simulink model "orbit_simulator"  (R2023a)
settings: Solver=ode4  StartTime=0.0  StopTime=5700  FixedStep=0.1  RelTol=1e-3
undefined symbols (not defined in the file or in its folder): X, Y, Z
libraries: robotlib x7, sharedtransform x6, aerolibutil x4, sharedutil x1
settings Model: Creator=yhj2019  LastModifiedBy=ohminsik
settings OptimizationCC: EnhancedBackFolding=on  PassReuseOutputArgsThreshold=0  MaxStackSize=64  OptimizeBlockOrder=speed  DifferentSizesBufferReuse=on  OptimizationCustomize=off
settings DebuggingCC: ParameterTunabilityLossMsg=error
settings HardwareCC: ProdBitPerPointer=32  ProdBitPerSizeT=32  ProdBitPerPtrDiffT=32  ProdLargestAtomicFloat=None  ProdIntDivRoundTo=Undefined  ProdEndianess=Unspecified  ProdWordSize=32  ProdHWDeviceType=Generic->Unspecified (assume 32-bit Generic)  UseEmbeddedCoderFeatures=off
settings SFSimCC: MATLABDynamicMemAlloc=off
settings RTWCC: Description=Embedded Coder  SystemTargetFile=ert.tlc  HardwareBoard=Robot Operating System (ROS)  TLCOptions="-aInlineSetEventsForThisBaseRateFcn=TLC_FALSE -aSuppressMultiTaskScheduler=TLC_FALSE  -aRateBasedStepFcn=0"  TemplateMakefile=ert_default_tmf  Toolchain=Catkin  TargetLang=C++
settings CodeAppCC: ForceParamTrailComments=on  OperatorAnnotations=on
settings ERTTargetCC: ERTCustomFileBanners=off  SupportContinuousTime=on  SupportNonInlinedSFcns=on  RemoveResetFunc=off  ModelStepFunctionPrototypeControlCompliant=off

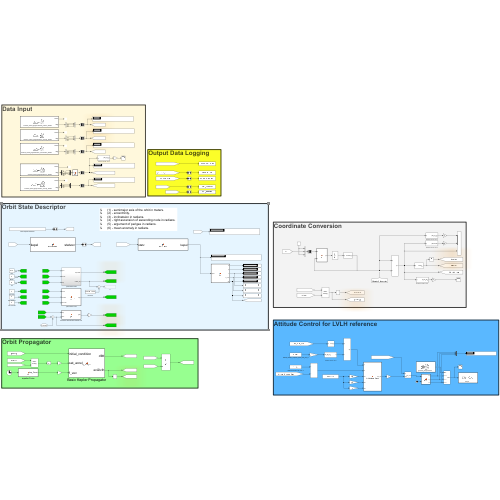
[thumbnail: Simulink's stored preview of the top-level diagram]
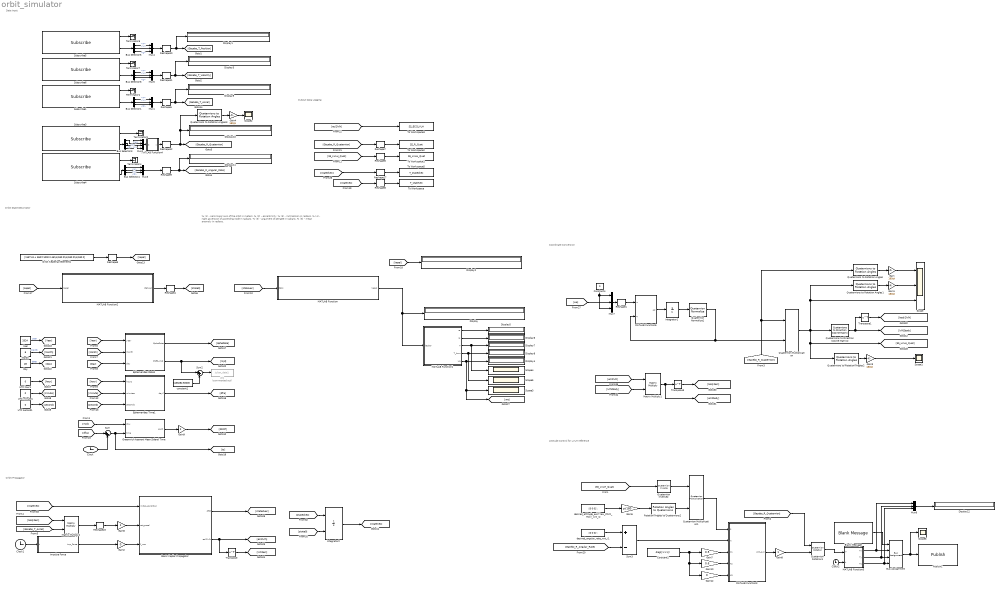
== system orbit_simulator ==
  note: Coordinate Conversion
  note: Orbit Propagator
  note: Output Data Logging
  note: Orbit State Descriptor
  note: Attitude Control for LVLH reference
  note: Data Input
  note: % (1) - semimajor axis of the orbit in meters.
      | % (2) - eccentricity.
      | % (3) - inclinatsion in radians.
      | % (4) - right ascension of ascending node in radians.
      | % (5) - argument of perigee in radians.
      | % (6) - mean anomaly in radians.
  Basic Kepler Propagator : MATLAB Function  TreatAsAtomicUnit=on
  Blank Message : robotlib/Blank Message  messageClass=Message  entityType=geometry_msgs/Vector3  messageType=geometry_msgs/Vector3  SampleTime=inf  legacyBusStruct=off
  Bus Assignment : BusAssignment  AssignedSignals=X,Y,Z
  Bus Selector{1,4..6} (4 alike) : BusSelector  OutputSignals=X,Y,Z
  Bus Selector3 : BusSelector  OutputSignals=X,Y,Z,W
  Clock : Clock
  Clock1 : Clock
  Clock2 : Clock
  Constant2 : Constant  Value=diag([1 1 1])
  Constant4 : Constant  Value=0
  Day : Constant  Value=28
  Display{,1..12} (13 alike) : Display
  Ephemerides Date1 : Subsystem
  Ephemerides Time1 : MATLAB Function  TreatAsAtomicUnit=on
  Gain{,1,3..4} (4 alike) : Gain  Gain=180/pi
  Gain10 : Gain  Gain=0.6
  Gain12 : Gain  Gain=0
  Gain2 : Gain  Gain=0
  Gain5 : Gain  Gain=pi/180
  Gain6 : Gain
  Gain7 : Gain  Gain=0.5
  Gain8 : Gain
  Gain9 : Gain
  Greenwich Aparent Mean Sideral Time : MATLAB Function  TreatAsAtomicUnit=on
  Impulse Force : MATLAB Function  TreatAsAtomicUnit=on
  Integrator1 : Integrator  InitialCondition=[1 0 0 0]'
  Integrator2 : Integrator  InitialConditionSource=external  InitialCondition=[-7000 0 0 0 -9.175045 0 5233.5]'
  JD1 : ToWorkspace  Commented=on  VariableName=Julian_date1  SampleTime=-1
  MATLAB Function : MATLAB Function  TreatAsAtomicUnit=on
  MATLAB Function1 : MATLAB Function  TreatAsAtomicUnit=on
  MATLAB Function2 : MATLAB Function  TreatAsAtomicUnit=on
  MATLAB Function3 : MATLAB Function  TreatAsAtomicUnit=on
  MATLAB Function4 : MATLAB Function  TreatAsAtomicUnit=on
  MATLAB Function5 : MATLAB Function  TreatAsAtomicUnit=on
  MATLAB Function6 : MATLAB Function  TreatAsAtomicUnit=on
  Matrix Multiply1 : Product  Multiplication=Matrix(*)
  Matrix Multiply2 : Product  Multiplication=Matrix(*)
  Month : Constant  Value=6
  Mux{1,3..7} (6 alike) : Mux  Inputs=3
  Mux2 : Mux
  Orbit Keplerian Elements : Constant  Value=[(6371.8 + 550)*1000 0 45*pi/180 0*pi/180 0*pi/180 0]
  Publish1 : robotlib/Publish  topicSource=Specify your own  topic=/torque  messageType=geometry_msgs/Vector3  legacyBusStruct=off  messageQueueLength=1
  Quaternion Inverse2 : aerolibutil/Quaternion Inverse
  Quaternion Multiplication : aerolibutil/Quaternion Multiplication
  Quaternion Multiplication1 : aerolibutil/Quaternion Multiplication
  Quaternion Normalize1 : sharedutil/Quaternion Normalize  aMode=aMode
  Quaternion Rotation1 : aerolibutil/Quaternion Rotation
  Quaternions to Direction Cosine Matrix2 : sharedtransform/Quaternions to  Direction Cosine Matrix  aMode=aMode
      settings: LibrarySourceBlock=|
      | aerolibtransform2/Quaternions to
      | Direction Cosine Matrix
  Quaternions to Rotation Angles : sharedtransform/Quaternions to Rotation Angles  rotationOrder=ZYX  aMode=aMode
  Quaternions to Rotation Angles1 : sharedtransform/Quaternions to Rotation Angles  rotationOrder=ZYX  aMode=aMode
  Quaternions to Rotation Angles2 : sharedtransform/Quaternions to Rotation Angles  rotationOrder=ZYX  aMode=aMode
  Quaternions to Rotation Angles3 : sharedtransform/Quaternions to Rotation Angles  rotationOrder=XYZ  aMode=aMode
  Reshape{1,5,9..12} (6 alike) : Reshape  OutputDimensionality=Column vector (2-D)
  Reshape{3..4,6..8,17} (6 alike) : Reshape  OutputDimensionality=Row vector (2-D)
  Reshape23 : Reshape  OutputDimensionality=Customize  OutputDimensions=[3,1]
  Rotation Angles to Quaternions2 : sharedtransform/Rotation Angles to Quaternions  rotationOrder=ZYX  aMode=aMode
  Scope : Scope  NumInputPorts=3
  Scope{1..6} (6 alike) : Scope
  Subscribe1 : robotlib/Subscribe  topicSource=Select from ROS network  topic=/reaction_wheel_plugin/transition_acceleration_throttle  messageType=geometry_msgs/Vector3  SampleTime=-1  legacyBusStruct=off  messageQueueLength=1
  Subscribe3 : robotlib/Subscribe  topicSource=Select from ROS network  topic=/reaction_wheel_plugin/quaternion_throttle  messageType=geometry_msgs/Quaternion  SampleTime=-1  legacyBusStruct=off  messageQueueLength=1
  Subscribe4 : robotlib/Subscribe  topicSource=Select from ROS network  topic=/reaction_wheel_plugin/rotation_velocity_throttle  messageType=geometry_msgs/Vector3  SampleTime=-1  legacyBusStruct=off  messageQueueLength=1
  Subscribe5 : robotlib/Subscribe  topicSource=Select from ROS network  topic=/reaction_wheel_plugin/transition_position_throttle  messageType=geometry_msgs/Vector3  SampleTime=-1  legacyBusStruct=off  messageQueueLength=1
  Subscribe6 : robotlib/Subscribe  topicSource=Select from ROS network  topic=/reaction_wheel_plugin/transition_velocity_throttle  messageType=geometry_msgs/Vector3  SampleTime=-1  legacyBusStruct=off  messageQueueLength=1
  Sum : Sum  Inputs=|++
  Sum2 : Sum  Inputs=|++
  Sum3 : Sum  Inputs=+-
  Terminator{1,3..4,6..7} (5 alike) : Terminator
  To Workspace : ToWorkspace  VariableName=T_statevec  SampleTime=-1
      settings: Save2DSignal=2-D array (concatenate along first dimension)
  To Workspace1 : ToWorkspace  VariableName=SS_LVLH_Quat  SampleTime=-1
      settings: Save2DSignal=2-D array (concatenate along first dimension)
  To Workspace2 : ToWorkspace  VariableName=SS_R_Quat  SampleTime=-1
      settings: Save2DSignal=2-D array (concatenate along first dimension)
  To Workspace3 : ToWorkspace  VariableName=SS_ECI2LVLH  SaveFormat=Structure With Time  SampleTime=-1
      settings: Save2DSignal=2-D array (concatenate along first dimension)
  To Workspace5 : ToWorkspace  VariableName=T_statedvec  SampleTime=-1
      settings: Save2DSignal=2-D array (concatenate along first dimension)
  Transpose : Math  Operator=transpose
  Transpose1 : Math  Operator=transpose
  Transpose3 : Math  Operator=transpose
  UTC hour1 : Constant  Value=0
  UTC minute1 : Constant  Value=0
  UTC second1 : Constant  Value=0
  Year : Constant  Value=2024
  constant1 : Constant  Value=2433282.50000
  desired_angular_rate_wrt_i1 : Constant  Value=[0 0 0]';
  desired_attitude_eulr(Yaw_Pitch_Roll)_wrt_i2 : Constant  Value=[0 0 0]';
  wires:
  MATLAB Function/1(kepel) -> Display/1, MATLAB Function1/1(kepler)
  Day/1 -> [Day]  "date"
  [statevec] -> Basic Kepler Propagator/1(initial_condition)
  Reshape3/1 -> [kepel]
  UTC hour1/1 -> [hour]
  Clock1/1 -> Impulse Force/1(t)
  MATLAB Function1/5(we) -> [we], Scope3/1, Display4/1
  Matrix Multiply2/1 -> Reshape23/1
  [minute] -> Ephemerides Time1/2(minutes)
  Reshape4/1 -> [state0]
  [statevec] -> Reshape8/1
  [kepel] -> MATLAB Function2/1(kepel)
  Clock/1 -> Sum/2
  MATLAB Function1/3(T) -> Scope4/1, Display7/1
  [Gazebo_T_Accel] -> Matrix Multiply2/2
  [statevec] -> MATLAB Function/1(statv)
  Basic Kepler Propagator/2(eci2lvlh) -> Transpose/1, [eci2lvlh]
  UTC minute1/1 -> [minute]
  Reshape8/1 -> To Workspace/1
  MATLAB Function1/1(ra) -> Display5/1
  [Year] -> Ephemerides Date1/1(year)
  [body2eci] -> Matrix Multiply2/1
  Month/1 -> [Month]  "month"
  Sum/1 -> Greenwich Aparent Mean Sideral Time/2(time), [ts]
  Basic Kepler Propagator/1(dfdt) -> [statedvec]
  Reshape17/1 -> To Workspace5/1
  [hour] -> Ephemerides Time1/1(hours)
  Gain6/1 -> Basic Kepler Propagator/2(sat_accel)
  MATLAB Function1/4(T_hour) -> Scope5/1, Display8/1
  Gain9/1 -> [GMST]
  Transpose/1 -> [lvlh2eci]
  [Month] -> Ephemerides Date1/2(month)
  Impulse Force/1(Imp_Force) -> Gain2/1
  MATLAB Function1/2(rp) -> Display6/1
  [Day] -> Ephemerides Date1/3(day)
  [statedvec] -> Reshape17/1
  [kepel] -> Display2/1
  UTC second1/1 -> [second]
  [second] -> Ephemerides Time1/3(seconds)
  [state0] -> Integrator2/2
  Sum2/1 -> JD1/1
  Gain2/1 -> Basic Kepler Propagator/3(f_vec)
  Ephemerides Date1/2(CNES_mdj) -> Sum2/1, [mjd]
  constant1/1 -> Sum2/2
  Reshape23/1 -> Gain6/1
  Integrator2/1 -> [statevec]
  Greenwich Aparent Mean Sideral Time/1(gwst) -> Gain9/1
  Ephemerides Date1/1(EpheDate) -> [EpheDate]
  Year/1 -> [Year]  "year"
  [statedvec] -> Integrator2/1
  MATLAB Function2/1(statvec) -> Reshape4/1
  Ephemerides Time1/1(dayf) -> [dfra]
  Orbit Keplerian Elements/1 -> Reshape3/1
  Subscribe5/2 -> Bus Selector5/1
  Bus Selector5/2 -> Mux4/2  "<Y>"
  Subscribe5/1 -> Terminator6/1
  Bus Selector5/3 -> Mux4/3  "<Z>"
  Bus Selector5/1 -> Mux4/1  "<X>"
  Mux4/1 -> Reshape10/1
  Reshape10/1 -> Display1/1, [Gazebo_T_Position]
  Bus Selector6/1 -> Mux5/1  "<X>"
  Bus Selector6/2 -> Mux5/2  "<Y>"
  Subscribe6/2 -> Bus Selector6/1
  Bus Selector6/3 -> Mux5/3  "<Z>"
  Subscribe6/1 -> Terminator7/1
  Mux5/1 -> Reshape11/1
  Reshape11/1 -> Display3/1, [Gazebo_T_Velocity]
  Bus Selector3/2 -> Mux2/3  "<Y>"
  Bus Selector3/4 -> Mux2/1  "<W>"
  Bus Selector3/1 -> Mux2/2  "<X>"
  Subscribe3/2 -> Bus Selector3/1
  Bus Selector3/3 -> Mux2/4  "<Z>"
  Subscribe3/1 -> Terminator3/1
  Mux2/1 -> MATLAB Function4/1(q)
  Bus Selector4/1 -> Mux3/1  "<X>"
  Mux3/1 -> Reshape9/1
  Bus Selector4/3 -> Mux3/3  "<Z>"
  Bus Selector4/2 -> Mux3/2  "<Y>"
  Subscribe4/1 -> Terminator4/1
  Subscribe4/2 -> Bus Selector4/1
  Reshape9/1 -> Display11/1, [Gazebo_R_Angular_Rate]
  Blank Message/1 -> Bus Assignment/1
  Bus Assignment/1 -> Scope6/1, Publish1/1
  Gain1/1 -> Scope/2
  Quaternion Multiplication/1 -> Quaternions to Direction Cosine Matrix2/1, [SS_LVLH_Quat], Quaternions to Rotation Angles2/1, Scope/3, Quaternions to Rotation Angles1/1
  Quaternion Normalize1/1 -> Quaternion Multiplication/2, MATLAB Function6/2(q)
  Quaternions to Rotation Angles1/1 -> Gain1/1
  Quaternions to Direction Cosine Matrix2/1 -> Transpose1/1, [lvlh2body]
  Quaternions to Rotation Angles/1 -> Gain/1
  Gain/1 -> Scope/1
  Transpose1/1 -> [body2lvlh]
  [Gazebo_R_Quaternion] -> Quaternion Multiplication/1, Quaternions to Rotation Angles/1
  MATLAB Function4/1(y) -> Reshape12/1
  Matrix Multiply1/1 -> Transpose3/1, [eci2body]
  Transpose3/1 -> [body2eci]
  [eci2lvlh] -> Matrix Multiply1/1
  [lvlh2body] -> Matrix Multiply1/2
  Subscribe1/2 -> Bus Selector1/1
  Subscribe1/1 -> Terminator1/1
  Bus Selector1/3 -> Mux1/3  "<Z>"
  Bus Selector1/1 -> Mux1/1  "<X>"
  Mux1/1 -> Reshape5/1
  Bus Selector1/2 -> Mux1/2  "<Y>"
  Reshape5/1 -> Display9/1, [Gazebo_T_Accel]
  Gain3/1 -> Scope1/1
  Quaternions to Rotation Angles2/1 -> Gain3/1
  Gain4/1 -> Scope2/1
  Quaternions to Rotation Angles3/1 -> Gain4/1
  Clock2/1 -> MATLAB Function5/2(t)
  MATLAB Function3/1(cntl_out) -> Gain8/1
  MATLAB Function5/3(Tz) -> Mux6/3, Bus Assignment/4
  MATLAB Function5/2(Ty) -> Mux6/2, Bus Assignment/3
  MATLAB Function5/1(Tx) -> Mux6/1, Bus Assignment/2
  Reshape6/1 -> To Workspace1/1
  [SS_LVLH_Quat] -> Reshape6/1
  [Gazebo_R_Quaternion] -> Reshape7/1
  Reshape7/1 -> To Workspace2/1
  [eci2lvlh] -> To Workspace3/1
  Reshape12/1 -> Quaternions to Rotation Angles3/1, Display10/1, [Gazebo_R_Quaternion]
  [Gazebo_R_Angular_Rate] -> Sum3/2
  Rotation Angles to Quaternions2/1 -> Quaternion Multiplication1/2
  Quaternion Inverse2/1 -> Quaternion Multiplication1/1
  Sum3/1 -> MATLAB Function3/2(w)
  Gain10/1 -> MATLAB Function3/4(K2)
  Gain7/1 -> MATLAB Function3/3(K1)
  Gain12/1 -> MATLAB Function3/5(K3)
  Constant2/1 -> Gain10/1, Gain12/1, Gain7/1
  Quaternion Multiplication1/1 -> MATLAB Function3/1(q)
  Gain5/1 -> Rotation Angles to Quaternions2/1
  desired_angular_rate_wrt_i1/1 -> Sum3/1
  desired_attitude_eulr(Yaw_Pitch_Roll)_wrt_i2/1 -> Gain5/1
  Constant4/1 -> Mux7/1, Mux7/3
  Reshape1/1 -> MATLAB Function6/1(w)
  Integrator1/1 -> Quaternion Normalize1/1
  MATLAB Function6/1(qd) -> Integrator1/1
  [we] -> Mux7/2
  Mux7/1 -> Reshape1/1
  [SS_LVLH_Quat] -> Quaternion Inverse2/1
  Gain8/1 -> Quaternion Rotation1/2
  Quaternion Rotation1/1 -> MATLAB Function5/1(T)
  [Gazebo_R_Quaternion] -> Quaternion Rotation1/1
  Mux6/1 -> Display12/1
  [mjd] -> Greenwich Aparent Mean Sideral Time/1(diju)
  [dfra] -> Sum/1

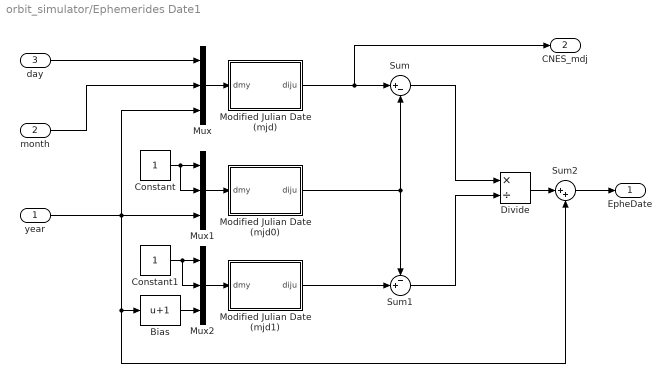
== system orbit_simulator/Ephemerides Date1 ==
  year : Inport
  month : Inport  Port=2
  day : Inport  Port=3
  Bias : Bias  Bias=1  SaturateOnIntegerOverflow=off
  Constant : Constant
  Constant1 : Constant
  Divide : Product  Inputs=*/
  Modified Julian Date (mjd) : MATLAB Function  TreatAsAtomicUnit=on
  Modified Julian Date (mjd0) : MATLAB Function  TreatAsAtomicUnit=on
  Modified Julian Date (mjd1) : MATLAB Function  TreatAsAtomicUnit=on
  Mux : Mux  Inputs=3
  Mux1 : Mux  Inputs=3
  Mux2 : Mux  Inputs=3
  Sum : Sum  Inputs=|+-
  Sum1 : Sum  Inputs=-+|
  Sum2 : Sum  Inputs=|++
  EpheDate : Outport
  CNES_mdj : Outport  Port=2
  wires:
  Sum1/1 -> Divide/2
  Modified Julian Date (mjd1)/1(diju) -> Sum1/2
  month/1 -> Mux/2
  year/1 -> Mux1/3, Mux/3, Bias/1, Sum2/2
  Mux1/1 -> Modified Julian Date (mjd0)/1(dmy)
  day/1 -> Mux/1
  Mux/1 -> Modified Julian Date (mjd)/1(dmy)
  Mux2/1 -> Modified Julian Date (mjd1)/1(dmy)
  Bias/1 -> Mux2/3
  Modified Julian Date (mjd)/1(diju) -> CNES_mdj/1, Sum/1
  Constant1/1 -> Mux2/2, Mux2/1
  Sum/1 -> Divide/1
  Constant/1 -> Mux1/2, Mux1/1
  Modified Julian Date (mjd0)/1(diju) -> Sum1/1, Sum/2
  Divide/1 -> Sum2/1
  Sum2/1 -> EpheDate/1

== matlab function orbit_simulator/MATLAB Function6 ==
  data: w input; q input; qd output
function qd = fcn(w, q)

w1 = w(1);
w2 = w(2);
w3 = w(3);

% Omega = [  0  -w1 -w2 -w3;
%                  w1     0   w3 -w2;
%                  w2 -w3     0   w1;
%                  w3   w2 -w1   0];
% q_v = [q(2), q(3), q(4)]';
% q_w = q(1);

% qd_v =-0.5*cross(w,q_v) + 0.5*q_w*w;
% qd_w = -0.5*w'*q_v;
% qd = [qd_w, qd_v(1), qd_v(2), qd_v(3)]';
Omega = [  0  w1  w2  w3;
         -w1   0 -w3  w2;
         -w2  w3   0 -w1;
         -w3 -w2  w1   0];
qd = -0.5*Omega*q;

end

== matlab function orbit_simulator/Ephemerides Date1/Modified Julian Date (mjd0) ==
  data: dmy input; diju output
function diju  =  djm (dmy)
% [diju] = djm (day, month, year)
%    The function djm furnishes the Modified Julian
%    Date with reference to the day, month and year,
%    at zero hours of the day.
% inputs:
%   dmy(1): day, day of the month
%   dmy(2): month, month of the year
%   dmy(3): year

% outputs:
%   diju
%       Modified Julian Date in days, referred to 1950.0. 
%
% Valdemir Carrara, Apr, 2003
%

diju = 367*dmy(3) + dmy(1) - 712269 + fix(275*dmy(2)/9)- fix(7*(dmy(3)+fix((dmy(2)+9)/12))/4);

== matlab function orbit_simulator/Ephemerides Date1/Modified Julian Date (mjd1) ==
  data: dmy input; diju output
function diju  =  djm (dmy)
% [diju] = djm (day, month, year)
%    The function djm furnishes the Modified Julian
%    Date with reference to the day, month and year,
%    at zero hours of the day.
% inputs:
%   dmy(1): day, day of the month
%   dmy(2): month, month of the year
%   dmy(3): year

% outputs:
%   diju
%       Modified Julian Date in days, referred to 1950.0. 
%
% Valdemir Carrara, Apr, 2003
%

diju = 367*dmy(3) + dmy(1) - 712269 + fix(275*dmy(2)/9)- fix(7*(dmy(3)+fix((dmy(2)+9)/12))/4);

== matlab function orbit_simulator/Ephemerides Time1 ==
  data: hours input; dayf output; minutes input; seconds input
function dayf  = time_to_dayf(hours, minutes, seconds)
% [dayf] = time_to_dayf (hours, minutes, seconds)
%    The function time_to_dayf returns with the day elapesed
%    time in seconds
% inputs:
%   hours     
%       day hour (integer).
%   minutes
%       minutes (integer).
%   seconds
%       seconds and fraction of second
% outputs:
%   dayf
%       Day elapsed time in seconds. 
%
% Valdemir Carrara, Feb, 2009
%

dayf = seconds + 60*(minutes + 60*hours);

== matlab function orbit_simulator/MATLAB Function ==
  data: statv input; kepel output
function kepel  = statvec_kepel (statv)
% [kepel] = statvec_kepel (statv)
%
%	The function statvec_kepel transforms the state vector statv
%	into the corresponding keplerian elements in the
%	same reference system.
%
% Input:
%	statv
%		state vector in meters and meters/second.
%
% Output:
%	statvec_kepel
%		vector containing the keplerian elements:
%		(1) - semimajor axis of the orbit in meters.
%		(2) - eccentricity.
%		(3) - inclination in radians.
%		(4) - right ascension of ascending node in radians.
%		(5) - argument of perigee in radians.
%		(6) - mean anomaly in radians.
%
% Authors:
%	Helio K. Kuga
%    Valder M. Medeiros
%	Valdemir Carrara			february/80			version 1.0
%	Helio K. Kuga     			august/82           version 2.0
%	Ulisses T V Guedes 			december/95	 		version 2.1
%               - fix perigee procedure when orbit plane
%                  equal to equatorial plane
%	Valdemir Carrara 			july/05				(C version)
%   Valdemir Carrara            March/09        Matlab

EARTH_GRAVITY	= 3.9860064e+14;		% Earth's gravitational constant (m**3/s**2)

xp  = [statv(1) statv(2) statv(3)];
xv  = [statv(4) statv(5) statv(6)];
r      = sqrt(xp*xp');
vq     = xv*xv';
ainv   = 2.0/r - vq/EARTH_GRAVITY;

h      = cross(xp, xv);
hm     = sqrt(h*h');
an = [0 0 0];
if (hm < 1.e-10)
    disp (' *** Message from function statvec_kepel: *** ');
    disp (' There are no keplerian elements corresponding to this state vector');
    kepel = [0, 0, 0, 0, 0, 0];
else
    h      = h/hm;
    incl   = acos(h(3));
    raan   = atan2(h(1), -h(2));
    d      = xp*xv' / EARTH_GRAVITY;
    esene  = d * sqrt(EARTH_GRAVITY*ainv);
    ecose  = 1 - r*ainv;
    exc    = sqrt(esene*esene + ecose*ecose);
    E      = atan2(esene, ecose);
    mean   = mod (E - esene, 2*pi);
    if mean < 0
        mean = mean + 2*pi;
    end

    if exc < 1.e-10
        arpe = 0;
    else
        dp     = 1./r - ainv;
        ev     = dp*xp - d*xv;
        abev   = sqrt(ev*ev');
        ev     = ev/abev;
        an(1)  = cos(raan);
        an(2)  = sin(raan);
        an(3)  = 0;
        fi     = ev*cross(h, an)';
        arpe = acos(ev*an');
        if fi < 0
            arpe  =  -arpe + 2*pi;
        end
    end

    kepel = [1./ainv, exc, incl, raan, arpe, mean];
end

end

== matlab function orbit_simulator/Basic Kepler Propagator ==
  data: initial_condition input; sat_accel input; dfdt output; f_vec input; eci2lvlh output
function [dfdt, eci2lvlh]   = eq_propagate(initial_condition, sat_accel, f_vec)

u  = 3.9865*10^14;
Re = 6378137; % earth radius in m
sat_mass = 100;%[kg]

dfdt = zeros(size(initial_condition));

x  = initial_condition(1); % x
y  = initial_condition(2); % y
z  = initial_condition(3); % z
x1 = initial_condition(4); % vel_x
y1 = initial_condition(5); % vel_y
z1 = initial_condition(6); % vel_z

r=sqrt(x^2+y^2+z^2);

% % %   Keplar Motion Equatnion
% % %  => r_dd + u/(r^3)r_ = 0 => r_dd = -u/(r^3)r_
dfdt(1) = x1;% vel_x
dfdt(2) = y1;% vel_y
dfdt(3) = z1;% vel_z
dfdt(4) = -u*x/r^3 + sat_accel(1) + f_vec(1)/sat_mass;% accel_x
dfdt(5) = -u*y/r^3 + sat_accel(2) + f_vec(2)/sat_mass;% accel_y
dfdt(6) = -u*z/r^3 + sat_accel(3) + f_vec(3)/sat_mass;% accel_z

% % % % % % % % % % % % LVLH Frame % % % % % % % % % % % % % % % % % % % % % % % % % % % % % % % % % % % %
% x as the unit vector directed along the spacecraft position vector:
lvlh_z = -[x;y;z]./r; 
% rcv    = cross([x;y;z],[x1;y1;z1]);
rcv    = [x1;y1;z1];
% z as the unit vector directed along the spacecraft's orbital angular momentum vector:
lvlh_x = rcv/norm(rcv);
% y as the unit vector that completes a right handed coordinate system:
lvlh_y = cross(lvlh_z, lvlh_x);

eci2lvlh = [lvlh_x, lvlh_y, lvlh_z];

end

== matlab function orbit_simulator/MATLAB Function2 ==
  data: kepel input; statvec output
function statvec  = kepel_statvec (kepel)
%  [statvec] = kepel_statvec (kepel)
%	The function kepel_statvec transforms the keplerian
%	elements kepel into the corresponding state vector in
%	the same reference system.
%
% Input:
%	kepel
% 		vector containing the keplerian elements:
%		(1) - semimajor axis of the orbit in meters.
%		(2) - eccentricity.
%		(3) - inclinatsion in radians.
%		(4) - right ascension of ascending node in radians.
%		(5) - argument of perigee in radians.
%		(6) - mean anomaly in radians.
% Output:
%	statvec
%  		state vector in meters and meters/second.
%
% Authors:
%	Helio K. Kuga;
%	Valder M. Medeiros;
%	Valdemir Carrara		february/80		version 1.0
%	Valdemir Carrara		july 2005		(C version)
%   Valdemir Carrara            March/09        Matlab

EARTH_GRAVITY	= 3.9860064e+14;		% Earth's gravitational constant (m**3/s**2)

a    = kepel(1);	% semi-major axis
exc  = kepel(2);	% eccentricity

c1   = sqrt(1. - exc*exc);

%     rotation matrix

orb2iner = rotmaz(-kepel(4))*rotmax(-kepel(3))*rotmaz(-kepel(5));

%     Kepler's equation

E    = kepler(kepel(6), exc);

sE   = sin(E);
cE   = cos(E);
c3   = sqrt(EARTH_GRAVITY/a)/(1. - exc*cE);

%     state vector

statvec = [[a*(cE - exc), a*c1*sE, 0]*orb2iner', [-c3*sE, c1*c3*cE, 0]*orb2iner'];

end

function [rot_mat] = rotmax (angle)
% [rot_mat] = rotmax (angle)
%   To obtain the rotation matrix around the X axis given the
%   rotation angle.
% inputs:
%   angle
%       rotation angle, in radians.
% outputs:
%   rot_mat
%       rotation matrix (3, 3)
%

% Valdemir Carrara, Sep, 1998

coan    =  cos(angle);
sian    =  sin(angle);

rot_mat =  [1, 0, 0; 0, coan, sian; 0, -sian, coan];

end

function [rot_mat] = rotmay (angle)
% [rot_mat] = rotmay (angle)
%   To obtain the rotation matrix around the Y axis given the
%   rotation angle.
% inputs:
%   angle
%       rotation angle, in radians.
% outputs:
%   rot_mat
%       rotation matrix (3, 3)
%

% Valdemir Carrara, Sep, 1998


coan    =  cos(angle);
sian    =  sin(angle);

rot_mat =  [coan, 0, -sian; 0, 1, 0; sian, 0, coan];

end

function [rot_mat] = rotmaz (angle)
% [rot_mat] = rotmaz (angle)
%   To obtain the rotation matrix around the Z axis given the
%   rotation angle.
% inputs:
%   angle
%       rotation angle, in radians.
% outputs:
%   rot_mat
%       rotation matrix (3, 3)
%

% Valdemir Carrara, Sep, 1998

coan    =  cos(angle);
sian    =  sin(angle);

rot_mat =  [coan, sian, 0; -sian, coan, 0; 0, 0, 1];
end

function [eccentric] = kepler (mean_anomaly, eccentricity)
% [eccentric] = kepler (mean_anomaly, eccentricity)
%	The subroutine kepler finds a solution to the
%	kepler's equation.
%
% Input:
%	mean_anomaly
%		mean anomaly in radians.
%	eccentricity
%		eccentricity.
%
% Output:
%	eccentric
%		eccentric anomaly in radians.
%
% Authors:
%	Valder M. de Medeiros		june/81		version 2.0
%	Valdemir Carrara			july 2005	(C version)
%   Valdemir Carrara            March/09        Matlab

exc2    = eccentricity*eccentricity;
am1     = mod (mean_anomaly, 2*pi);
am2     = am1 + am1;
am3     = am1 + am2;
shoot   = am1 + eccentricity*(1. - 0.125*exc2)*sin(am1) + ...
		0.5*exc2*(sin(am2) + 0.75*eccentricity*sin(am3));
shoot   = mod (shoot, 2*pi);

e1      = 1.0;
ic      = 0;

while ((abs(e1) > 1.e-12) && (ic <= 10)) 
	e1    = (shoot - am1 - eccentricity*sin(shoot)) / ...
			(1.0 - eccentricity*cos(shoot));
    shoot = shoot - e1;
    ic    = ic + 1;
end

if (ic >= 10)
    disp ('warning ** subroutine kepler did not converge in 10 iterations');
end

eccentric = shoot;


end

== matlab function orbit_simulator/MATLAB Function1 ==
  data: kepler input; ra output; rp output; T output; T_hour output; we output
function [ra, rp, T, T_hour, we] = fcn(kepler)

u=3.9865*10^14;

a = kepler(1);
e = kepler(2);
% 

ra = a*(1+e);%장반경
rp = a*(1-e);%단반경

a = (ra+rp)/2;% semi-major axis

% a = (550 + 6371.8)*1000;

T = 2*pi*sqrt((a*a*a)/(u));

T_hour = T/3600;

we = 2*pi/T;
% we = 1.1207*0.001;

end

== matlab function orbit_simulator/Impulse Force ==
  settings: updateMethod=DISCRETE
  data: Imp_Force output; t input
function Imp_Force  = fcn(t)

Imp_Force = [0 0 0]';

if ((t >= 1000) && (t <= 1050))
    Imp_Force =  [-10000 0 10000]';
elseif ((t >= 1100) && (t <= 1150))
    Imp_Force = -[-20000 0 10000]';
else
    Imp_Force = [0 0 0]';

end

end

== matlab function orbit_simulator/MATLAB Function4 ==
  data: q input; y output
function y = fcn(q)

if ((q(1) == 0) && (q(2) == 0) && (q(3) == 0) && (q(4) == 0))
    y = [1 0 0 0]';
else
    y = q;
end

end

== matlab function orbit_simulator/MATLAB Function5 ==
  data: T input; t input; Tx output; Ty output; Tz output
function [Tx, Ty, Tz] = fcn(T, t)

if(t<=10)
 Tx = 0;
 Ty = 0;
 Tz = 0;
else
 Tx = T(1);
 Ty = T(2);
 Tz = T(3);
end

T = [Tx,Ty,Tz]';
end

== matlab function orbit_simulator/Greenwich Aparent Mean Sideral Time ==
  data: diju input; gwst output; time input
function gwst  = gst (diju, time)
% [gwst] = gst (diju, time)
%   The function gst furnishes the greenwich aparent mean 
%   sidereal time referred to the J2000.0 equator and equinox.
% inputs:
%   diju
%       Modified Julian Date in days, referred to 1950.0.
%   time
%       UT1 time complement in seconds.
% outputs:
%   gwst
%       Greenwich aparent sidereal time in radians
%
% Valdemir Carrara, Apr, 2003
%

tsj = (diju-18262.5)/36525;
tsgo = (24110.54841 + (8640184.812866 + 9.3104e-2*tsj - 6.2e-6*tsj*tsj)*tsj)*pi/43200;
tetp = 7.292116e-5;		% velocidade angular da Terra (rd/s) mean angular velocity of the Earth
gwst = mod(tsgo + time*tetp, 2*pi);
% reference site
% https://www2.mps.mpg.de/homes/fraenz/systems/systems2art/node10.html
%      if (gwst<0) gwst = gwst + 2*pi

== matlab function orbit_simulator/MATLAB Function3 ==
  settings: updateMethod=DISCRETE
  data: q input; cntl_out output; w input; K1 input; K2 input; K3 input
function cntl_out = LVLH_Attitude_Control(q, w, K1, K2, K3)

persistent flg
persistent I_save

dt = 0.01;

if isempty(flg)
    flg = 1;
    I_save = [0 0 0]';
end

qs = q(1);
qv = [q(2), q(3), q(4)]';
w  = [w(1), w(2), w(3)]';

% K1 = diag([0.05 0.05 0.05]);
% K2 = diag([0.4 0.4 0.4]);

cntl_out = (sign(qs)*K1*qv + K2*w + K3*I_save);

I_save = I_save + dt*qv;


end

== matlab function orbit_simulator/Ephemerides Date1/Modified Julian Date (mjd) ==
  data: dmy input; diju output
function diju  =  djm (dmy)
% [diju] = djm (day, month, year)
%    The function djm furnishes the Modified Julian
%    Date with reference to the day, month and year,
%    at zero hours of the day.
% inputs:
%   dmy(1): day, day of the month
%   dmy(2): month, month of the year
%   dmy(3): year

% outputs:
%   diju
%       Modified Julian Date in days, referred to 1950.0. 
%
% Valdemir Carrara, Apr, 2003
%

diju = 367*dmy(3) + dmy(1) - 712269 + fix(275*dmy(2)/9)- fix(7*(dmy(3)+fix((dmy(2)+9)/12))/4);
